simulink model "Rudder_system_control2020_5"  (R2022b)
settings: Solver=VariableStepAuto  StartTime=0.0  StopTime=1800  MaxStep=0.02  RelTol=1e-3  AbsTol=1e-3  EnableMultiTasking=on
model workspace (MAT data in the model file):
  lowerLimitSaturation = -0.1
  upperLimitSaturation = 0.1
values from neighbouring files (symbols this model uses):
  Fg = 1    [start.m]
  H = 1    [start.m]
  Js = 1    [start.m]
  PistonStroke = 0.6    [start.m]
undefined symbols (not defined in the file or in its folder): sigbuilder_block
libraries: fl_lib x71, nesl_utility x16, sh_lib x2, simulink x1, aerolibconvert2 x1
(part 1 of 2)
CloseFcn:
  | try,close(h1_ssc_hydraulic_actuator_analog_control),end
  | clear h1_ssc_hydraulic_actuator_analog_control
  | 
  | clear simlog_ssc_hydraulic_actuator_analog_control
Description:
  | Hydraulic Actuator with Analog Position Controller
settings Model: Creator=MathWorks  LastModifiedBy=matheusassis
settings SolverCC: AutoScaleAbsTol=off  AlgebraicLoopSolver=LineSearch
settings DataIOCC: LimitDataPoints=on  SaveFormat=Array  ReturnWorkspaceOutputs=off
settings OptimizationCC: LifeSpan=inf
settings DebuggingCC: SolverPrmCheckMsg=warning  UnconnectedInputMsg=warning  UnconnectedOutputMsg=warning  UnconnectedLineMsg=warning  AllowSymbolicDim=off  PregeneratedLibrarySubsystemCodeDiagnostic=none  SFUnexpectedBacktrackingDiag=warning  SFNoUnconditionalDefaultTransitionDiag=warning  SFExecutionAtInitializationDiag=none  SFMachineParentedDataDiag=warning  ArithmeticOperatorsInVariantConditions=warning
settings HardwareCC: ProdBitPerPointer=32  ProdBitPerSizeT=32  ProdBitPerPtrDiffT=32  ProdLargestAtomicFloat=None  ProdIntDivRoundTo=Undefined  ProdEndianess=Unspecified  ProdWordSize=32  ProdHWDeviceType=32-bit Generic
settings ModelReferenceCC: EnableRefExpFcnMdlSchedulingChecks=on  PropagateSignalLabelsOutOfModel=off
settings SFSimCC: SimUseLocalCustomCode=off  CustomCodeUndefinedFunction=UseInterfaceOnly
settings RTWCC: RTWUseLocalCustomCode=off
settings CodeAppCC: StateflowObjectComments=on
settings GRTTargetCC: TargetLangStandard=C89/C90 (ANSI)
settings ConfigComp: CovMetricSettings=dw  CovSaveCumulativeToWorkspaceVar=on  CovSaveSingleToWorkspaceVar=on  CovExternalEMLEnable=off  CovSFcnEnable=off
settings SimscapeCC: SimscapeLogType=all  SimscapeLogSimulationStatistics=on  SimscapeLogName=simlog_ssc_hydraulic_actuator_analog_control  SimscapeLogDataHistory=10000

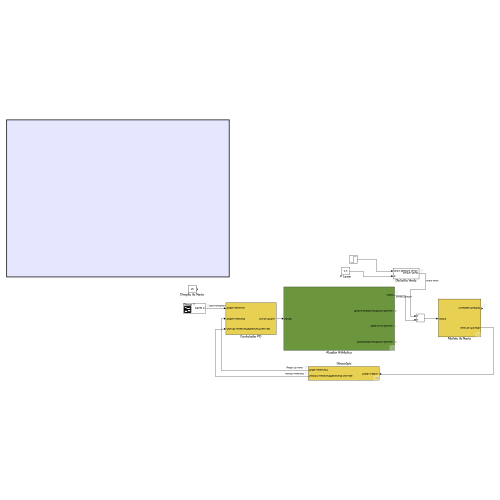
[thumbnail: Simulink's stored preview of the top-level diagram]
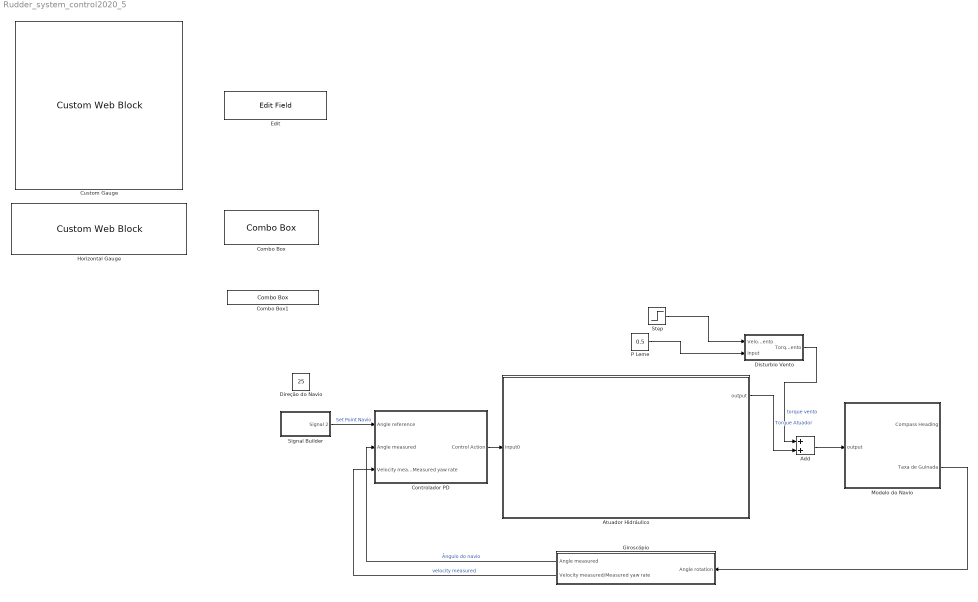
== system Rudder_system_control2020_5 ==
  " Giroscópio" : Subsystem
  Add : Sum
  Atuador Hidráulico : Subsystem
  Combo Box : ComboBox  SelectedLabel=20
      settings: Values={{'30', '20', '10'}, [0.5 0.35 0.18]}
  Combo Box1 : ComboBox  LabelPosition=Hide  SelectedLabel=Normal
      settings: Values={{'Normal', 'Mau Tempo'}, [18 40]}
  Controlador PD : Subsystem
  Custom Gauge : CustomWebBlock  Configuration="{\"components\":[{\"name\":\"CircularScaleComponent\",\"settings\":{\"bounds\":{\"max\":180,\"min\":-180,\"tickInterval\":\"auto\"},\"direction\":\"cw\",\"flipLimits\":0,\"innerRadius\":0.4437938380012364,\"internalTickHeightScaleFactor\":1,\"labelColor\":[250,245,200],\"labelFont\":{\"font\":\"Arial\",\"fontSize\":12},\"labelRadius\":0.36,\"labelTransparency\":1,\"minorTickHeightScaleFactor\":0.2,\"needleImage\":{\"size\":[0,0],\"src\":\"data:image\\/svg+xml;base64,PD94bWwgdmVyc2lvbj0iMS4wIiBlbmNvZGluZz0idXRmLTgiPz4KPCEtLSBHZW5lcmF0b3I6IEFkb2JlIElsbHVzdHJhdG9yIDE5LjIuMSwgU1ZHIEV4cG9ydCBQbHVnLUluIC4gU1ZHIFZlcnNpb246IDYuMDAgQnVpbGQgMCkgIC0tPgo8c3ZnIHZlcnNpb249IjEuMSIgeG1sbnM9Imh0dHA6Ly93d3cudzMub3JnLzIwMDAvc3ZnIiB4bWxuczp4bGluaz0iaHR0cDovL3d3dy53My5vcmcvMTk5OS94bGluayIgeD0iMHB4IiB5PSIwcHgiCgkgdmlld0JveD0iMCAwIDIwMCA1MCIgc3R5bGU9ImVuYWJsZS1iYWNrZ3JvdW5kOm5ldyAw ...(+9940 chars)\"},\"needleOffset\":[0.08810590036800516,0],\"needleOrientation\":-45,\"needleRotation\":-180,\"needleSize\":{\"height\":null,\"width\":0.3656531968792428},\"outerRadius\":0.5958029544034255,\"position\":[0,0,1,1],\"referencePoint\":\"auto\",\"scaleAngle\":299.999999999988,\"scaleAngleOffset\":119.46147497096791,\"scaleColors\":[{\"Color\":[0,0.44705882352941173,0.7411764705882353],\"Max\":0,\"Min\":0}],\"scaleColorsSize\":0.2,\"scaleDirection\":\"CW\",\"scalePosition\":[0,0,1,1],\"showLabels\":1,\"showMinorTicks\":1,\"showSpanLine\":1,\"showTicks\":1,\"tickColor\":[250,245,200],\"tickTransparency\":1,\"valueBarColor\":[23,89,176],\"valueBarPosition\":[0,0,1,1],\"valueBarSize\":0.2,\"valueBarTransparency\":1}},{\"name\":\"BackgroundImageComponent\",\"settings\":{\"image\":{\"size\":[0,0],\"src\":\"data:image\\/svg+xml;base64,PD94bWwgdmVyc2lvbj0iMS4wIiBlbmNvZGluZz0iVVRGLTgiIHN0YW5kYWxvbmU9Im5vIj8+CjwhLS0gR2VuZXJhdG9yOiBBZG9iZSBJbGx1c3RyYXRvciAxOS4yLjEsIFNWRyBFeHBvcnQgUGx1Zy1JbiAuIFNWRyBWZXJzaW9uOiA2LjAwIEJ1aWxkIDApICAtLT4KCjxzdmcKICAgeG1sbnM6ZGM9Imh0dHA6Ly9wdXJsLm9yZy9kYy9lbGVtZW50cy8xLjEvIgogICB4bWxuczpjYz0iaHR0cDovL2NyZWF0aXZlY29tbW9ucy5vcmcvbnMjIgogICB4bWxuczpyZGY9Imh0dHA6Ly93d3cudzMub3JnLzE5OTkvMDIvMjItcmRmLXN5bnRh ...(+9660 chars)\",\"srcOrientation\":\"horizontal\"},\"position\":[0,0,1,1],\"scaleMode\":\"0\"}},{\"name\":\"ForegroundImageComponent\",\"settings\":{\"image\":{\"size\":[0,0],\"src\":\"default\",\"srcOrientation\":[]},\"isForeground\":1,\"position\":[0,0,1,1],\"scaleMode\":\"0\"}}],\"settings\":{\"BindingType\":\"signal\",\"backgroundOffset\":0.14,\"backgroundOpacity\":1,\"fixedAspectRatio\":\"on\",\"orientation\":\"horizontal\",\"showBackgroundColor\":0},\"type\":\"CircularGauge\"}"
  Direção do Navio : Constant  Value=25
  Disturbio Vento : Subsystem
  Edit : EditField  ShowInitialText=on  Alignment=Center
  Horizontal Gauge : CustomWebBlock  ShowInitialText=on  Configuration="{\"components\":[{\"name\":\"LinearScaleComponent\",\"settings\":{\"bounds\":{\"max\":35,\"min\":-35,\"tickInterval\":\"auto\"},\"labelColor\":[250,245,199],\"labelFont\":{\"font\":\"Arial\",\"fontSize\":12},\"labelOffset\":0.05,\"labelTransparency\":1,\"needleImage\":{\"size\":[21,75],\"src\":\"data:image\\/svg+xml;base64,PHN2ZyB4bWxucz0iaHR0cDovL3d3dy53My5vcmcvMjAwMC9zdmciIHhtbG5zOnhsaW5rPSJodHRwOi8vd3d3LnczLm9yZy8xOTk5L3hsaW5rIiB2aWV3Qm94PSIwIDAgMjEgNzUiPjxkZWZzPjxzdHlsZT4uY2xzLTF7ZmlsbDpub25lO30uY2xzLTJ7aXNvbGF0aW9uOmlzb2xhdGU7fS5jbHMtM3tjbGlwLXBhdGg6dXJsKCNjbGlwLXBhdGgpO30uY2xzLTR7b3BhY2l0eTowLjM7bWl4LWJsZW5kLW1vZGU6bXVsdGlwbHk7fS5jbHMtNXtmaWxsOiNlYjI2Mjk7fTwvc3R5bGU+PGNsaXBQYXRoIGlkPSJjbGlwLXBhdGgiIHRyYW5zZm9y ...(+1928 chars)\",\"srcOrientation\":\"Right\"},\"needleOffset\":[0,0.01094391244870041],\"needleSize\":{\"height\":0.7589285714285714,\"width\":0.11960078534031414},\"position\":[0.06986607142857143,0.01995798319327731,0.9641544117647058,0.8],\"referencePoint\":\"auto\",\"scaleColorSize\":0.24,\"scaleColors\":[],\"scaleColorsSize\":0.2,\"scaleDirection\":\"LR\",\"tickColor\":[250,245,200],\"tickTransparency\":1,\"valueBarColor\":[23,89,176],\"valueBarSize\":0.23,\"valueBarTransparency\":1}},{\"name\":\"BackgroundImageComponent\",\"settings\":{\"image\":{\"size\":[380,101],\"src\":\"data:image\\/svg+xml;base64,PHN2ZyB4bWxucz0iaHR0cDovL3d3dy53My5vcmcvMjAwMC9zdmciIHhtbG5zOnhsaW5rPSJodHRwOi8vd3d3LnczLm9yZy8xOTk5L3hsaW5rIiB2aWV3Qm94PSIwIDAgMzgwIDEwMSI+PGRlZnM+PHN0eWxlPi5jbHMtMXtmaWxsOnVybCgjbGluZWFyLWdyYWRpZW50KTt9LmNscy0ye2ZpbGw6dXJsKCNsaW5lYXItZ3JhZGllbnQtMik7fS5jbHMtM3tmaWxsOnVybCgjbGluZWFyLWdyYWRpZW50LTMpO308L3N0eWxlPjxsaW5lYXJHcmFkaWVudCBpZD0ibGluZWFyLWdyYWRpZW50IiB5MT0iNTAuNSIgeDI9IjM5OS4yOCIgeTI9IjUw ...(+2216 chars)\",\"srcOrientation\":\"horizontal\"},\"position\":[0,0,1,1],\"scaleMode\":\"0\"}}],\"settings\":{\"BindingType\":\"signal\",\"fixedAspectRatio\":\"on\",\"orientation\":\"horizontal\"},\"type\":\"LinearGauge\"}"
  Modelo do Navio : Subsystem
  P Leme : Constant  Value=0.5
  Signal Builder : Subsystem  Tag=STV Subsys  LoadFcn=sigbuilder_block('load');  StartFcn=sigbuilder_block('start');  StopFcn=sigbuilder_block('stop');  ClipboardFcn=sigbuilder_block('clipboard');  mask(Sigbuilder block){tuvar=[0:10]}
      mask help: Simulink:masks:SigbuilderBlock_MD
      mask init:
      | if ~strcmp(get_param(bdroot(gcbh),'SimulationStatus'),'stopped') tuvar = sigbuilder_block('maskInit'); end
      settings: CopyFcn=sigbuilder_block('copy');  DeleteFcn=sigbuilder_block('delete');  ModelCloseFcn=sigbuilder_block('modelClose');  PreSaveFcn=sigbuilder_block('preSave');  PauseFcn=sigbuilder_block('pause');  ContinueFcn=sigbuilder_block('continue');  NameChangeFcn=sigbuilder_block('namechange');  OpenFcn=sigbuilder_block('open',[437.6 199.2 550.4 400 ]);  CloseFcn=sigbuilder_block('close');
      mask Display: plot(0, 0, 100, 100,[2, 2, 32, 32, 2], [68, 8, 8, 68, 68],[32, 2], [38, 38], [32, 19, 2],[53, 60, 44], [32, 17, 17, 2],[16, 16, 31, 31]);txt = getActiveGroup(gcbh);text(2, 100, txt,'verticalAlignment', 'top');
  Step : Step  After=50  SampleTime=0
  wires:
  Controlador PD/1(Control Action) -> Atuador Hidráulico/1(input0)
  Modelo do Navio/2(Taxa de Guinada) -> " Giroscópio"/1(Angle rotation)
  " Giroscópio"/1(Angle measured) -> Controlador PD/2(Angle measured)  "Ângulo do navio"
  " Giroscópio"/2(Velocity measured/Measured yaw rate) -> Controlador PD/3(Velocity measured/Measured yaw rate)  "velocity measured"
  Step/1 -> Disturbio Vento/1(Veloc Relativa Vento)
  P Leme/1 -> Disturbio Vento/2(Input)
  Atuador Hidráulico/1(output) -> Add/2  "Torque Atuador"
  Signal Builder/1(Signal 2) -> Controlador PD/1(Angle reference)  "Set Point Navio"
  Disturbio Vento/1(Torque Vento) -> Add/1  "torque vento"
  Add/1 -> Modelo do Navio/1(output)

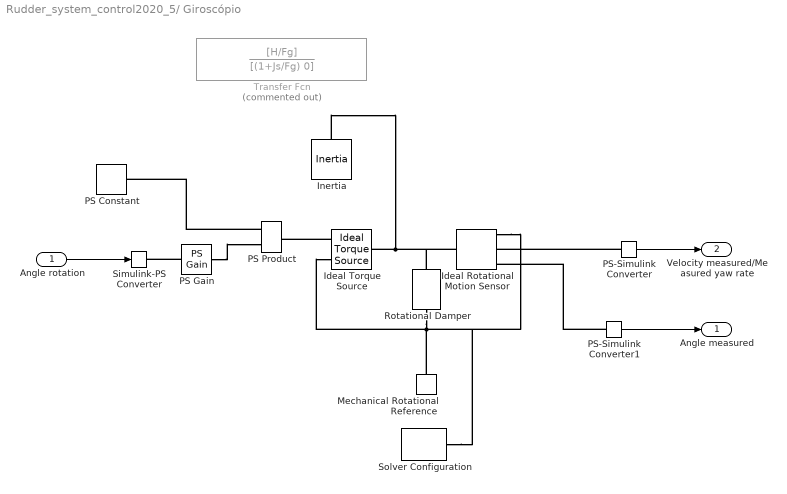
== system Rudder_system_control2020_5/ Giroscópio ==
  Angle rotation : Inport
  Ideal Rotational Motion Sensor : fl_lib/Mechanical/Mechanical Sensors/Ideal Rotational Motion Sensor  reference=foundation.enum.MeasurementReference.difference  acceleration_port=false  velocity_port=true  position_port=true  wrap_angle=simscape.enum.onoff.off  offset=0 rad
  Ideal Torque Source : fl_lib/Mechanical/Mechanical Sources/Ideal Torque Source
  Inertia : fl_lib/Mechanical/Rotational Elements/Inertia  inertia=0.08 kg*m^2  num_ports=foundation.enum.numPorts2.one  w_specify=off  w_priority=High  w=0 rad/s  w_nominal_specify=off  w_nominal_unit=rad/s  w_nominal_value=1  t_specify=off  t_priority=None  t=0 N*m  t_nominal_specify=off  t_nominal_unit=N*m  t_nominal_value=1
  Mechanical Rotational Reference : fl_lib/Mechanical/Rotational Elements/Mechanical Rotational Reference
  PS Constant : fl_lib/Physical Signals/Sources/PS Constant  constant=1
  PS Gain : fl_lib/Physical Signals/Functions/PS Gain  gain=0.017
  PS Product : fl_lib/Physical Signals/Functions/PS Product
  PS-Simulink Converter : nesl_utility/PS-Simulink Converter  PhysicalDomain=network_engine_domain  SubClassName=ps_output  LeftPortType=input  RightPortType=output  PseudoPeriodic=off  Frequencies=[]  VectorFormat=1-D array  Unit=inherit  AffineConversion=off
  PS-Simulink Converter1 : nesl_utility/PS-Simulink Converter  PhysicalDomain=network_engine_domain  SubClassName=ps_output  LeftPortType=input  RightPortType=output  PseudoPeriodic=off  Frequencies=[]  VectorFormat=1-D array  Unit=inherit  AffineConversion=off
  Rotational Damper : fl_lib/Mechanical/Rotational Elements/Rotational Damper  D=2 N*m/(rad/s)  w_specify=off  w_priority=None  w=0 rad/s  w_nominal_specify=off  w_nominal_unit=rad/s  w_nominal_value=1  t_specify=off  t_priority=None  t=0 N*m  t_nominal_specify=off  t_nominal_unit=N*m  t_nominal_value=1
  Simulink-PS Converter : nesl_utility/Simulink-PS Converter  PhysicalDomain=network_engine_domain  SubClassName=ps_input  LeftPortType=input  RightPortType=output  PseudoPeriodic=off  Frequencies=[]  NoiseDistribution=none  NoiseParameters=[]  Unit=1  AffineConversion=off  FilteringAndDerivatives=provide  SimscapeFilterOrder=1  InputFilterTimeConstant=0.001  UdotUserProvided=0
  Solver Configuration : nesl_utility/Solver Configuration  PhysicalDomain=network_engine_domain  SubClassName=solver  LeftPortType=input  RightPortType=generic  Tones=[]  Harmonics=[]  SimulateNoise=off  Profile=off  UseLocalSampling=off  EnableSwitchedLinearOptims=on  FrequencyDomain=off  UseCCode=off  RelTol=0.001  AbsTol=1e-06  MinStep=1e-09  ToWorkspace=off  RevertToSquareIcSolve=off  NumHomotopyIterations=100  PhasorMode=off  PhasorModeNumHarmonics=1  ConsistencySolver=NEWTON_FTOL  IndexReductionMethod=DerivativeReplacement  DoDC=off  ResidualTolerance=1e-09  ConsistencyTolSource=GLOBAL  ConsistencyAbsTol=0.001  ConsistencyRelTol=0.001  ConsistencyTolFactor=0.001  UseLocalSolver=off  LocalSolverChoice=NE_BACKWARD_EULER_ADVANCER  ResolveIndetEquations=on  FunctionEvalNumThread=1  LocalSolverSampleTime=0.001  DoFixedCost=off  MaxNonlinIter=3  MaxModeIter=2  ComputeImpulses=off  ImpulseIterations=2  LinearAlgebra=auto  LinearAlgebraNumThread=0  EquationFormulation=NE_TIME_EF  DelaysMemoryBudget=1024  AutomaticFiltering=on  FilteringTimeConstant=0.001  PartitionStorageMethod=AS_NEEDED  PartitionMemoryBudget=1024  PartitionMethod=ROBUST
  Transfer Fcn : TransferFcn  Commented=on  Numerator=[H/Fg]  Denominator=[(1+Js/Fg) 0]
  Angle measured : Outport
  Velocity measured/Measured yaw rate : Outport  Port=2
  wires:
  Angle rotation/1 -> Simulink-PS Converter/1
  PS-Simulink Converter/1 -> Velocity measured/Measured yaw rate/1
  PS-Simulink Converter1/1 -> Angle measured/1
  connections:
  PS Product/LConn1 -- PS Constant/RConn1
  PS Gain/LConn1 -- Simulink-PS Converter/RConn1
  PS Gain/RConn1 -- PS Product/LConn2
  Ideal Torque Source/RConn1 -- PS Product/RConn1
  Mechanical Rotational Reference/LConn1 -- Ideal Torque Source/RConn2 -- Rotational Damper/RConn1 -- Solver Configuration/RConn1 -- Ideal Rotational Motion Sensor/RConn1
  Inertia/LConn1 -- Rotational Damper/LConn1 -- Ideal Rotational Motion Sensor/LConn1 -- Ideal Torque Source/LConn1
  PS-Simulink Converter/LConn1 -- Ideal Rotational Motion Sensor/RConn2
  PS-Simulink Converter1/LConn1 -- Ideal Rotational Motion Sensor/RConn3

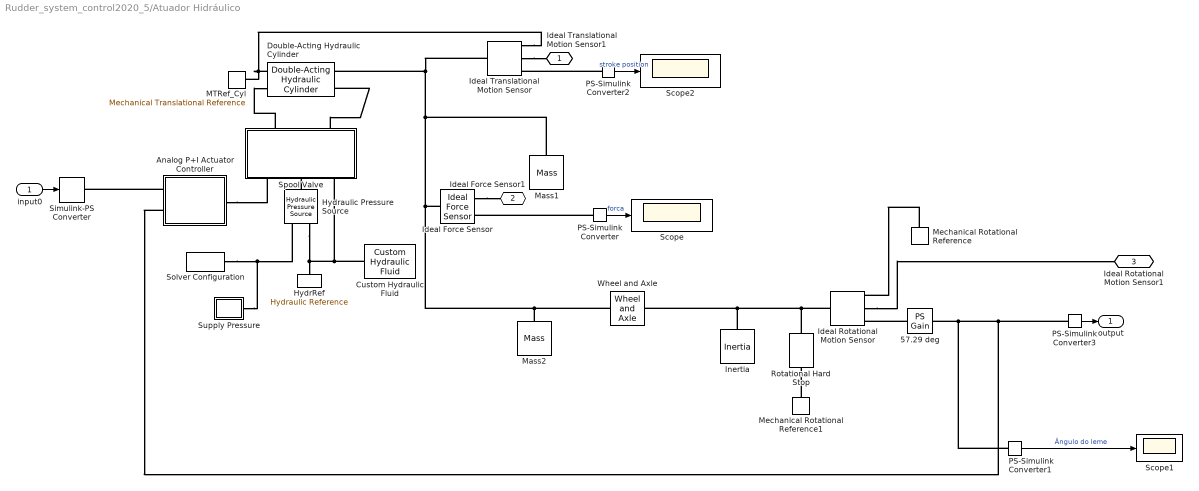
== system Rudder_system_control2020_5/Atuador Hidráulico ==
  input0 : Inport
  57.29 deg : fl_lib/Physical Signals/Functions/PS Gain  gain=57.29 deg
  Analog P+I Actuator Controller : Subsystem
  Custom Hydraulic Fluid : fl_lib/Hydraulic/Hydraulic Utilities/Custom Hydraulic Fluid  density=850 kg/m^3  viscosity_kin=1.8e-05 m^2/s  bulk=8e+08 Pa  alpha=0.005  range_error=2
      settings: InternalSimscapePortConfiguration="{\"Bottom\":[],\"Left\":[],\"Right\":[{\"id\":\"G\",\"label\":\"\",\"type\":\"foundation.hydraulic.hydraulic\"}],\"Top\":[]}"
  Double-Acting Hydraulic Cylinder : sh_lib/Hydraulic Cylinders/Double-Acting Hydraulic Cylinder  area_A=PistonArea m^2  area_B=PistonArea m^2  stroke=PistonStroke*2 m  dead_vol_A=1e-4 m^3  dead_vol_B=1e-4 m^3  k_sh=1.4  or=1  stiff=1e6 N/m  D=150 N/(m/s)  hardstop_model=1  transition=0.1 mm  displacement_spec=foundation.enum.DisplacementSpec.Calculate  init_pos=PistonStroke m  init_pressure_A=0 Pa  init_pressure_B=0 Pa
      settings: InternalSimscapePortConfiguration="{\"Bottom\":[],\"Left\":[{\"id\":\"C\",\"label\":\"C\",\"type\":\"foundation.mechanical.translational.translational\"},{\"id\":\"A\",\"label\":\"A\",\"type\":\"foundation.hydraulic.hydraulic\"}],\"Right\":[{\"id\":\"R\",\"label\":\"R\",\"type\":\"foundation.mechanical.translational.translational\"},{\"id\":\"B\",\"label\":\"B\",\"type\":\"foundation.hydraulic.hydraulic\"}],\"Top\":[]}"
  HydrRef : fl_lib/Hydraulic/Hydraulic Elements/Hydraulic Reference
  Hydraulic Pressure Source : fl_lib/Hydraulic/Hydraulic Sources/Hydraulic Pressure Source
      settings: InternalSimscapePortConfiguration="{\"Bottom\":[],\"Left\":[{\"id\":\"P\",\"label\":\"P\",\"type\":\"foundation.hydraulic.hydraulic\"}],\"Right\":[{\"id\":\"S\",\"label\":\"S\",\"type\":\"input\"},{\"id\":\"T\",\"label\":\"T\",\"type\":\"foundation.hydraulic.hydraulic\"}],\"Top\":[]}"
  Ideal Force Sensor : fl_lib/Mechanical/Mechanical Sensors/Ideal Force Sensor
  Ideal Rotational Motion Sensor : fl_lib/Mechanical/Mechanical Sensors/Ideal Rotational Motion Sensor  reference=foundation.enum.MeasurementReference.difference  acceleration_port=false  velocity_port=true  position_port=true  wrap_angle=simscape.enum.onoff.off  offset=0 deg
  Ideal Translational Motion Sensor : fl_lib/Mechanical/Mechanical Sensors/Ideal Translational Motion Sensor  reference=foundation.enum.MeasurementReference.difference  acceleration_port=false  velocity_port=true  position_port=true  offset=0 m
  Inertia : fl_lib/Mechanical/Rotational Elements/Inertia  inertia=Izz kg*m^2  num_ports=foundation.enum.numPorts2.one  w_specify=off  w_priority=High  w=0 rad/s  w_nominal_specify=off  w_nominal_unit=rad/s  w_nominal_value=1  t_specify=off  t_priority=None  t=0 N*m  t_nominal_specify=off  t_nominal_unit=N*m  t_nominal_value=1
  MTRef_Cyl : fl_lib/Mechanical/Translational Elements/Mechanical Translational Reference
  Mass1 : fl_lib/Mechanical/Translational Elements/Mass  mass=PistonMass kg  num_ports=foundation.enum.numPorts2.one  v_specify=off  v_priority=High  v=0 m/s  v_nominal_specify=off  v_nominal_unit=m/s  v_nominal_value=1  f_specify=off  f_priority=High  f=0 N  f_nominal_specify=off  f_nominal_unit=N  f_nominal_value=1
  Mass2 : fl_lib/Mechanical/Translational Elements/Mass  mass=1000 kg  num_ports=foundation.enum.numPorts2.one  v_specify=off  v_priority=High  v=0 m/s  v_nominal_specify=off  v_nominal_unit=m/s  v_nominal_value=1  f_specify=off  f_priority=High  f=0 N  f_nominal_specify=off  f_nominal_unit=N  f_nominal_value=1
  Mechanical Rotational Reference : fl_lib/Mechanical/Rotational Elements/Mechanical Rotational Reference
  Mechanical Rotational Reference1 : fl_lib/Mechanical/Rotational Elements/Mechanical Rotational Reference
  PS-Simulink Converter{,1..3} (4 alike) : nesl_utility/PS-Simulink Converter  PhysicalDomain=network_engine_domain  SubClassName=ps_output  LeftPortType=input  RightPortType=output  PseudoPeriodic=off  Frequencies=[]  VectorFormat=1-D array  Unit=inherit  AffineConversion=off
  Rotational Hard Stop : fl_lib/Mechanical/Rotational Elements/Rotational Hard Stop  upper_bnd=30 deg  lower_bnd=-30 deg  stiff_up=1e6 N*m/rad  stiff_low=1e6 N*m/rad  D_up=0.01 N*m/(rad/s)  D_low=0.01 N*m/(rad/s)  model=simscape.enum.hardstop.smooth  transition=0.001 rad  w_specify=off  w_priority=None  w=0 rad/s  w_nominal_specify=off  w_nominal_unit=rad/s  w_nominal_value=1  t_specify=off  t_priority=None  t=0 N*m  t_nominal_specify=off  t_nominal_unit=N*m  t_nominal_value=1  phi_specify=off  phi_priority=High  phi=0 rad  phi_nominal_specify=off  phi_nominal_unit=rad  phi_nominal_value=1
  Scope : Scope
  Scope1 : Scope
  Scope2 : Scope
  Simulink-PS Converter : nesl_utility/Simulink-PS Converter  PhysicalDomain=network_engine_domain  SubClassName=ps_input  LeftPortType=input  RightPortType=output  PseudoPeriodic=off  Frequencies=[]  NoiseDistribution=none  NoiseParameters=[]  Unit=V  AffineConversion=off  FilteringAndDerivatives=zero  SimscapeFilterOrder=1  InputFilterTimeConstant=.001  UdotUserProvided=0
  Solver Configuration : nesl_utility/Solver Configuration  PhysicalDomain=network_engine_domain  SubClassName=solver  LeftPortType=input  RightPortType=generic  Tones=[]  Harmonics=[]  SimulateNoise=off  Profile=off  UseLocalSampling=off  EnableSwitchedLinearOptims=on  FrequencyDomain=off  UseCCode=off  RelTol=0.001  AbsTol=1e-06  MinStep=1e-09  ToWorkspace=off  RevertToSquareIcSolve=off  NumHomotopyIterations=100  PhasorMode=off  PhasorModeNumHarmonics=1  ConsistencySolver=NEWTON_FTOL  IndexReductionMethod=DerivativeReplacement  DoDC=off  ResidualTolerance=1e-9  ConsistencyTolSource=GLOBAL  ConsistencyAbsTol=0.001  ConsistencyRelTol=0.001  ConsistencyTolFactor=0.001  UseLocalSolver=off  LocalSolverChoice=NE_BACKWARD_EULER_ADVANCER  ResolveIndetEquations=on  FunctionEvalNumThread=1  LocalSolverSampleTime=0.001  DoFixedCost=off  MaxNonlinIter=3  MaxModeIter=2  ComputeImpulses=off  ImpulseIterations=2  LinearAlgebra=auto  LinearAlgebraNumThread=0  EquationFormulation=NE_TIME_EF  DelaysMemoryBudget=1024  AutomaticFiltering=on  FilteringTimeConstant=0.001  PartitionStorageMethod=AS_NEEDED  PartitionMemoryBudget=1024  PartitionMethod=ROBUST
  Spool Valve : Subsystem  Tag=PublishSubsystem  mask(Single-Stage Servo Valve){K_V=0.5, x_max=0.5, A_max=9, x_lap=0.02, A_leak=0.25, G=0.5e-3/(pi/2), J=1e-4, lambda=0.01, R=10, L=2.5, Kt=0.04, R_controller=[10e3 10e3 10e3 100e3 50 100e3 10e3]}
      mask prompts: K_V "Flow Coefficient:"; x_max "Spool displacement limit (mm)"; A_max "Maximum orifice area (mm^2)"; x_lap "Spool displacement range for leakage (mm)"; A_leak "Leakage area at x=0 (mm^2)"; G "Spool displacement per motor rotation (m/radian)"; J "Total inertia reflected to motor (kg m^2)"; lambda "Total damping reflected to motor (Nm/(rad/s))"; R "Torque motor winding resistance (ohms)"; L "Torque motor winding inductance (H)"; Kt "Torque motor torque constant (Nm/A)"; R_controller "Motor controller resistance values [R1 R2 R3 R4 R5 R6 R7] (ohms)"
      mask help: Models a spool valve actuated directly by a torque motor.
      mask Display:
      | % Plot icon
      | plot([0;337.311462499201;337.311462499201;0;0], [566.910021007061;566.910021007061;0;0;566.910021007061])
      | plot([84.6585631370544;241.503668949008], [353;353])
      | plot([84.6585631370544;241.503668949008], [214;214])
      | plot([84.6585631370544;241.503668949008;241.503668949008;84.6585631370544;84.6585631370544], [491;491;76;76;491])
      | plot([84.6585631370544;241.503668949008], [449;449])
      | plot([241.503668949008;210.071657784283], [310;310])
      | plot([210.071657784283;210.071657784283;210.071657784283], [326;295;310.414731502533])
      | plot([241.503668949008;210.071657784283], [257;257])
      | plot([210.071657784283;210.071657784283;210.071657784283], [272;241;236.464468762279])
      | plot([84.6585631370544;115.964594297111], [257;257])
      | plot([115.964594297111;115.964594297111;115.964594297111], [272;241;236.464468762279])
      | plot([84.6585631370544;115.964594297111], [310;310])
      | plot([115.964594297111;115.964594297111;115.964594297111], [326;295;310.414731502533])
      | plot([84.6585631370544;241.503668949008], [185;110])
      | plot([241.503668949008;84.6585631370544], [185;110])
      | plot([84.6585631370544;241.503668949008], [395;395])
      | patch([85.0365031510592;110.547454096377;121.885654516518;85.0365031510592], [110;140;120;110], [0;0;0])
      | plot([85.0365031510592;110.547454096377;121.885654516518;85.0365031510592], [110;140;120;110])
      | patch([240.936758928001;204.087607562542;215.425807982683;240.936758928001], [109;120;140;109], [0;0;0])
      | 
      | plot([240.936758928001;204.087607562542;215.425807982683;240.936758928001], [109;120;140;109])
      | patch([83.6507230997086;127.554754726589;127.554754726589;83.6507230997086], [394;405;384;394], [0;0;0])
      | plot([83.6507230997086;127.554754726589;127.554754726589;83.6507230997086], [394;405;384;394])
      | patch([245.283069089055;201.253057457507;201.253057457507;245.283069089055], [451;461;440;451], [0;0;0])
      | plot([245.283069089055;201.253057457507;201.253057457507;245.283069089055], [451;461;440;451])
      | 
      | % Port labels
      | color('red')
      | port_label('LConn', 1,'S')
      | port_label('LConn', 2,'P')
      | port_label('LConn', 3,'T')
      | port_label('RConn', 1,'A')
      | port_label('RConn', 2,'B')
      | color('black')
  Supply Pressure : Subsystem
  Wheel and Axle : fl_lib/Mechanical/Mechanisms/Wheel and Axle  R=1.30 m  or=1  t_specify=off  t_priority=None  t=0 N*m  t_nominal_specify=off  t_nominal_unit=N*m  t_nominal_value=1  f_specify=off  f_priority=None  f=0 N  f_nominal_specify=off  f_nominal_unit=N  f_nominal_value=1
  Ideal Translational Motion Sensor1 : PMIOPort  Side=Right
  Ideal Force Sensor1 : PMIOPort  Port=2  Side=Right
  Ideal Rotational Motion Sensor1 : PMIOPort  Port=3  Side=Right
  output : Outport
  wires:
  PS-Simulink Converter/1 -> Scope/1  "forca"
  PS-Simulink Converter1/1 -> Scope1/1  "Ângulo do leme"
  PS-Simulink Converter2/1 -> Scope2/1  "stroke position"
  input0/1 -> Simulink-PS Converter/1
  PS-Simulink Converter3/1 -> output/1
  connections:
  Custom Hydraulic Fluid/RConn1 -- Hydraulic Pressure Source/RConn2 -- HydrRef/LConn1 -- Spool Valve/LConn3
  Ideal Force Sensor/LConn1 -- Mass1/LConn1 -- Ideal Translational Motion Sensor/LConn1 -- Double-Acting Hydraulic Cylinder/RConn1 -- Wheel and Axle/RConn1 -- Mass2/LConn1
  Double-Acting Hydraulic Cylinder/LConn1 -- MTRef_Cyl/LConn1 -- Ideal Translational Motion Sensor/RConn1
  Analog P+I Actuator Controller/LConn2 -- PS-Simulink Converter1/LConn1 -- 57.29 deg/RConn1 -- PS-Simulink Converter3/LConn1
  Spool Valve/RConn2 -- Double-Acting Hydraulic Cylinder/RConn2
  Analog P+I Actuator Controller/LConn1 -- Simulink-PS Converter/RConn1
  Supply Pressure/RConn1 -- Solver Configuration/RConn1 -- Hydraulic Pressure Source/RConn1
  Mechanical Rotational Reference1/LConn1 -- Rotational Hard Stop/RConn1
  Inertia/LConn1 -- Ideal Rotational Motion Sensor/LConn1 -- Rotational Hard Stop/LConn1 -- Wheel and Axle/LConn1
  57.29 deg/LConn1 -- Ideal Rotational Motion Sensor/RConn3
  Mechanical Rotational Reference/LConn1 -- Ideal Rotational Motion Sensor/RConn1
  Ideal Force Sensor/RConn1 -- Ideal Force Sensor1/RConn1
  Hydraulic Pressure Source/LConn1 -- Spool Valve/LConn2
  PS-Simulink Converter/LConn1 -- Ideal Force Sensor/RConn2
  Spool Valve/RConn1 -- Double-Acting Hydraulic Cylinder/LConn2
  Analog P+I Actuator Controller/RConn1 -- Spool Valve/LConn1
  PS-Simulink Converter2/LConn1 -- Ideal Translational Motion Sensor/RConn3
  Ideal Rotational Motion Sensor/RConn2 -- Ideal Rotational Motion Sensor1/RConn1
  Ideal Translational Motion Sensor/RConn2 -- Ideal Translational Motion Sensor1/RConn1
